simulink model "twoaxis_camera_gantry_start"  (R2021b)
settings: Solver=VariableStepAuto  StartTime=0.0  StopTime=inf  MaxStep=0.01  RelTol=1e-3  AbsTol=0.001  EnableMultiTasking=on
model workspace: external: MATLAB File gantryParams.m (data not in the file)
values from neighbouring files (symbols this model uses):
  endSupport = struct    [gantryParams.m]
  endSupportZ = struct    [gantryParams.m]
  leadScrew = struct    [gantryParams.m]
  leadScrewZ = struct    [gantryParams.m]
  rail = struct    [gantryParams.m]
  railZ = struct    [gantryParams.m]
  runner = struct    [gantryParams.m]
  runnerZ = struct    [gantryParams.m]
undefined symbols (not defined in the file or in its folder): DiscIntNeverNeededParam, X, Y, Z
libraries: sm_lib x81, nesl_utility x30, fl_lib x26, sm_linear_actuator_lib x14, ee_lib x4, slpidlib x2, mspsensorlib x1
(part 1 of 5)
Description:
  | Using the Lead Screw Joint Block - Linear Actuator
  | 
  | This example illustrates the use of the Lead Screw Joint block to model a linear actuator. The Lead
  | Screw Joint block converts rotational motion at the Revolute Joint block to translational motion at
  | the four Cylindrical Joint blocks. The translational motion is specified as a motion input to a
  | cylindrical joint and the necessary actuator torque is automatically computed at the revolute joint.
settings Model: Creator=The MathWorks, Inc.  LastModifiedBy=mligu
settings SolverCC: MaxConsecutiveZCs=100  ZeroCrossAlgorithm=Adaptive  AlgebraicLoopSolver=TrustRegion
settings DataIOCC: SaveFormat=Array  ReturnWorkspaceOutputsName=tp63adcd96_f5aa_4336_8232_618a6ec8fe4f  Refine=20
settings OptimizationCC: LifeSpan=inf
settings DebuggingCC: MaxConsecutiveZCsMsg=none  SolverPrmCheckMsg=warning  AllowSymbolicDim=off  ModelReferenceExtraNoncontSigs=warning  StateNameClashWarn=warning  SFUnexpectedBacktrackingDiag=warning  SFNoUnconditionalDefaultTransitionDiag=warning  SFExecutionAtInitializationDiag=none  SFMachineParentedDataDiag=warning  ArithmeticOperatorsInVariantConditions=warning
settings ModelReferenceCC: PropagateSignalLabelsOutOfModel=off
settings SFSimCC: SimUseLocalCustomCode=off  CustomCodeUndefinedFunction=UseInterfaceOnly
settings RTWCC: RTWUseLocalCustomCode=off
settings CodeAppCC: StateflowObjectComments=on
settings GRTTargetCC: TargetLangStandard=C89/C90 (ANSI)
settings ConfigComp: CovMetricSettings=dw  CovSaveCumulativeToWorkspaceVar=on  CovSaveSingleToWorkspaceVar=on  CovExternalEMLEnable=off  CovSFcnEnable=off
settings SimscapeCC: SimscapeNormalizeSystem=off
settings ConfigurationSet: Description=SimMechanics 2G
settings DiagnosticsConfigSet: SimMechanicsUnconnectedFramePorts=none
settings ExplorerConfigSet: InternalSimMechanicsExplorerSettings="<ExplorerConfiguration><canonicalview>default</canonicalview><AnimationSetting><BasePlaybackSpeed>1.0</BasePlaybackSpeed><PlaybackSpeedFactor>1.0</PlaybackSpeedFactor></AnimationSetting><TilePanel><TileInfo><Tiles Columns=\"1\" Count=\"1\" Rows=\"1\"><Column Weight=\"1\"/><Row Weight=\"1\"/><Tile Height=\"1\" Width=\"1\" X=\"0\" Y=\"0\"/></Tiles></TileInfo><SceneInfo><SceneViewer><BGColor><R>1</R><G>1</G><B>1</B></BGColor><Camera><DoPerspective>off</DoPerspective><Position><X>0.577350260811389404</X><Y>-0.277350261388458308</Y><Z>0.937350262073923357</Z></Position><Center><X>-8.37823641020030152e-09</X><Y>0.300000007801167534</Y><Z>0.35999999288429757</Z></Center><Up><X>-0.408248290463863073</X><Y>0.408248290463863073</Y><Z>0.816496580927726145</Z></Up><ViewLimDist>1</ViewLimDist><YLim>0.483570086956024159</YLim><XLim>0.367001870038164535</XLim></Camera></SceneViewer></SceneInfo></TilePanel><MechEditorPanel><Cameras/><GfxPanelCameraMap/><VideoCreator><PlaybackSpeedRatio>1.0</PlaybackSpeedRatio><FrameRate>30</FrameRate><VideoFormat>Motion JPEG AVI</VideoFormat><FrameSize>auto</FrameSize></VideoCreator></MechEditorPanel></ExplorerConfiguration>"

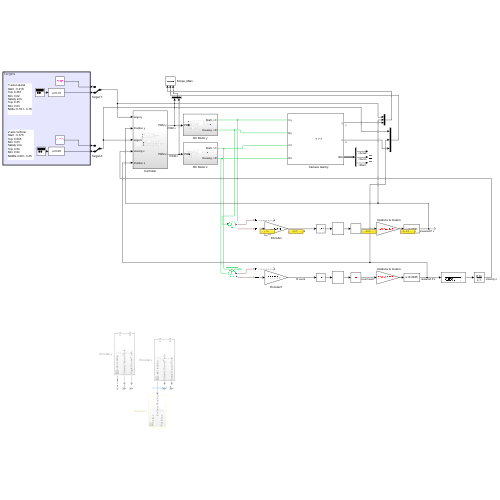
[thumbnail: Simulink's stored preview of the top-level diagram]
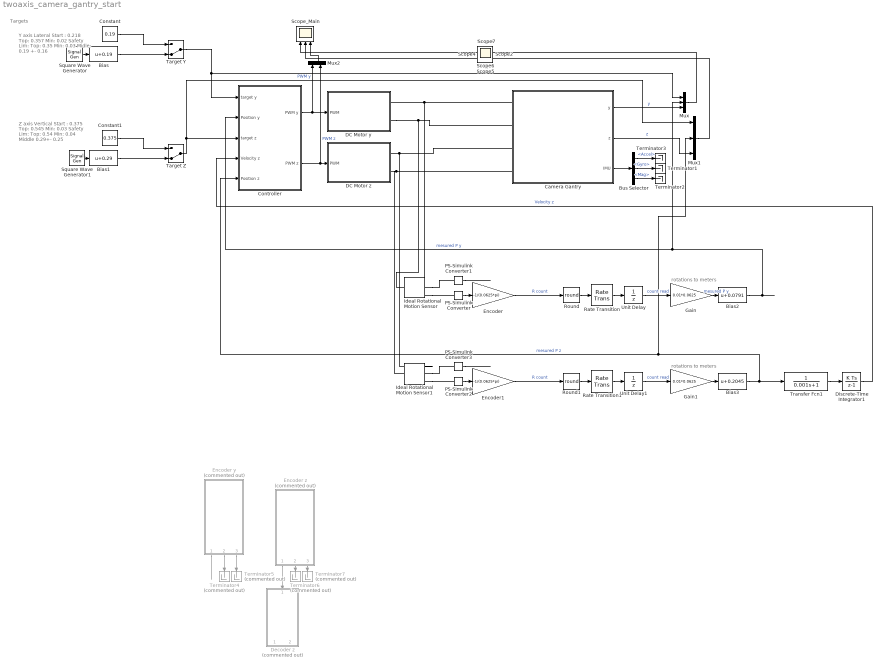
== system twoaxis_camera_gantry_start ==
  note: rotations to meters
  note: Z axis Vertical
      | Start : 0.375
      | Top: 0.545
      | Min: 0.03
      | Safety Lim:
      | Top: 0.54
      | Min: 0.04
      | Middle 0.29+- 0.25
  note: Targets
  note: Y axis Lateral
      | Start : 0.218
      | Top: 0.357
      | Min: 0.02
      | Safety Lim:
      | Top: 0.35
      | Min: 0.03
      | Midle: 0.19 +- 0.16
  note: rotations to meters
  "\tCamera Gantry" : Subsystem
      mask Display: image('C:\Users\cirie\Documents\MCT_labs\coursework_individual\camera_gantry\images\camera_gantry.png'); % Use "Edit Image" on toolstrip to change.
  Bias : Bias  Bias=0.19
  Bias1 : Bias  Bias=0.29
  Bias2 : Bias  Bias=0.0791
  Bias3 : Bias  Bias=0.2045
  Bus Selector : BusSelector  OutputSignals=Accel,Gyro,Mag
  Constant : Constant  Value=0.19
  Constant1 : Constant  Value=0.375
  Controller : Subsystem
  DC Motor y : Subsystem
  DC Motor z : Subsystem
  Decoder z : Subsystem  Commented=on
  Discrete-Time Integrator1 : DiscreteIntegrator  SampleTime=-1  ICPrevOutput=DiscIntNeverNeededParam  ICPrevScaledInput=DiscIntNeverNeededParam
  Encoder : Gain  Gain=-1/(0.0625*pi)
  Encoder y : Subsystem  Commented=on
  Encoder z : Subsystem  Commented=on
  Encoder1 : Gain  Gain=-1/(0.0625*pi)
  Gain : Gain  Gain=0.01*0.0625
  Gain1 : Gain  Gain=0.01*0.0625
  Ideal Rotational Motion Sensor : fl_lib/Mechanical/Mechanical Sensors/Ideal Rotational Motion Sensor  wrap_angle=simscape.enum.onoff.off  offset=0 rad
  Ideal Rotational Motion Sensor1 : fl_lib/Mechanical/Mechanical Sensors/Ideal Rotational Motion Sensor  wrap_angle=simscape.enum.onoff.off  offset=0 rad
  Mux : Mux  Inputs=3
  Mux1 : Mux  Inputs=3
  Mux2 : Mux  Inputs=2
  PS-Simulink Converter{,1..3} (4 alike) : nesl_utility/PS-Simulink Converter  PhysicalDomain=network_engine_domain  SubClassName=ps_output  LeftPortType=input  RightPortType=output  PseudoPeriodic=off  Frequencies=[]  Unit=inherit  AffineConversion=off
      settings: SourceProductBaseCode=PW,SS
  Rate Transition : RateTransition
  Rate Transition1 : RateTransition
  Round : Rounding  Operator=round
  Round1 : Rounding  Operator=round
  Scope_Main : Scope  NumInputPorts=3
  Square Wave Generator : SignalGenerator  Amplitude=0.16  Frequency=0.5  Units=rad/sec
  Square Wave Generator1 : SignalGenerator  Amplitude=0.25  Frequency=0.6  Units=rad/sec
  Target Y : ManualSwitch  CurrentSetting=0
  Target Z : ManualSwitch  CurrentSetting=0
  Terminator1 : Terminator
  Terminator2 : Terminator
  Terminator3 : Terminator
  Terminator{4..7} (4 alike) : Terminator  Commented=on
  Transfer Fcn1 : TransferFcn  Denominator=[0.001 1]
  Unit Delay : UnitDelay  SampleTime=-1  HasFrameUpgradeWarning=on
  Unit Delay1 : UnitDelay  SampleTime=-1  HasFrameUpgradeWarning=on
  Scope{,1..2,4..7} (7 alike) : Scope
  wires:
  "\tCamera Gantry"/3(IMU) -> Bus Selector/1
  Bus Selector/2 -> Terminator1/1  "<Gyro>"
  Bus Selector/3 -> Terminator2/1  "<Mag>"
  "\tCamera Gantry"/2(z) -> Mux1/3  "z"
  Controller/1(PWM y) -> Mux2/1, DC Motor y/1(PWM)  "PWM y"
  Controller/2(PWM z) -> Mux2/2, DC Motor z/1(PWM)  "PWM z"
  Square Wave Generator/1 -> Bias/1
  Square Wave Generator1/1 -> Bias1/1
  Bias/1 -> Target Y/2
  Target Z/1 -> Controller/3(target z), Mux1/1
  Bias1/1 -> Target Z/2
  Constant1/1 -> Target Z/1
  Constant/1 -> Target Y/1
  Target Y/1 -> Controller/1(target y), Mux/1
  Mux/1 -> Scope_Main/1
  Mux1/1 -> Scope_Main/2
  Mux2/1 -> Scope_Main/3
  Bus Selector/1 -> Terminator3/1  "<Accel>"
  Encoder y/1(Encoder reading) -> ?
  Encoder z/1(Encoder reading) -> Decoder z/1(Encoder Reading)
  "\tCamera Gantry"/1(y) -> Mux/3  "y"
  Encoder y/2(Velocity Ground Truth) -> Terminator4/1
  Encoder y/3(Angle Ground Truth) -> Terminator5/1
  Encoder z/2(Velocity Ground Truth) -> Terminator6/1
  Encoder z/3(Angle Ground Truth) -> Terminator7/1
  Bias2/1 -> Controller/2(Position y), Mux/2  "mesured P y"
  Unit Delay/1 -> Gain/1  "count read"
  Encoder/1 -> Round/1  "R count"
  PS-Simulink Converter1/1 -> ?
  Rate Transition/1 -> Unit Delay/1
  Round/1 -> Rate Transition/1
  PS-Simulink Converter/1 -> Encoder/1
  Bias3/1 -> Mux1/2, Controller/5(Position z), Transfer Fcn1/1  "mesured P z"
  Unit Delay1/1 -> Gain1/1  "count read"
  PS-Simulink Converter2/1 -> Encoder1/1
  Encoder1/1 -> Round1/1  "R count"
  Transfer Fcn1/1 -> Discrete-Time Integrator1/1
  PS-Simulink Converter3/1 -> ?
  Round1/1 -> Rate Transition1/1
  Rate Transition1/1 -> Unit Delay1/1
  Discrete-Time Integrator1/1 -> Controller/4(Velocity z)  "Velocity z"
  Gain/1 -> Bias2/1  "mesured P y"
  Gain1/1 -> Bias3/1
  connections:
  "\tCamera Gantry"/LConn3 -- Ideal Rotational Motion Sensor1/RConn1 -- DC Motor z/RConn1
  "\tCamera Gantry"/LConn1 -- Ideal Rotational Motion Sensor/RConn1 -- DC Motor y/RConn1
  DC Motor y/RConn2 -- Ideal Rotational Motion Sensor/LConn1 -- "\tCamera Gantry"/LConn2
  "\tCamera Gantry"/LConn4 -- Ideal Rotational Motion Sensor1/LConn1 -- DC Motor z/RConn2
  Ideal Rotational Motion Sensor/RConn3 -- PS-Simulink Converter/LConn1
  Ideal Rotational Motion Sensor/RConn2 -- PS-Simulink Converter1/LConn1
  Ideal Rotational Motion Sensor1/RConn3 -- PS-Simulink Converter2/LConn1
  Ideal Rotational Motion Sensor1/RConn2 -- PS-Simulink Converter3/LConn1

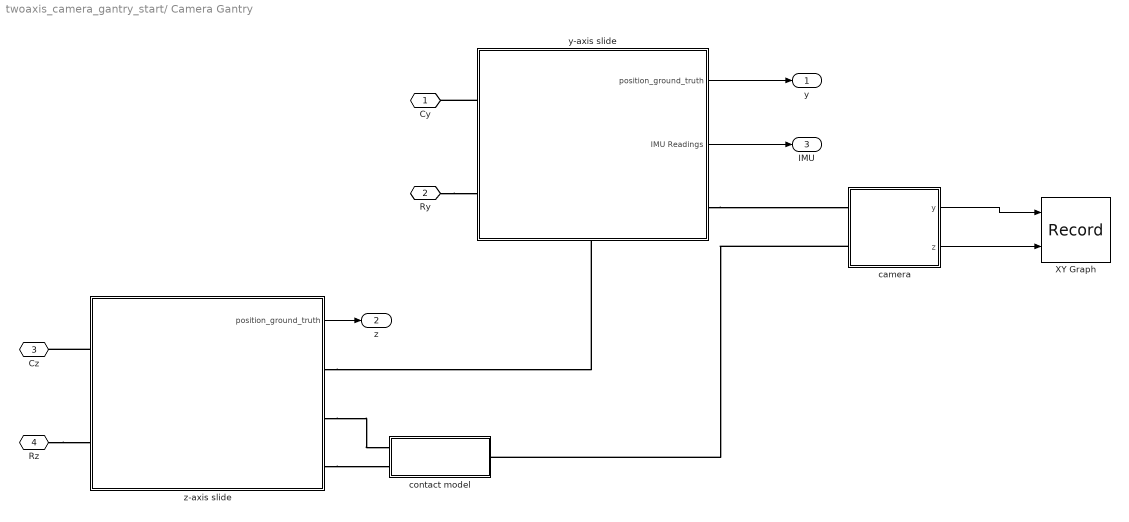
== system twoaxis_camera_gantry_start/	Camera Gantry ==
  XY Graph : Record  FileSettingsInternal="{\"entries\":[{\"content\":{\"excelSettings\":{\"content\":{},\"type\":\"Streamout.ExcelSettings\"}},\"type\":\"Streamout.FileSettingStorage\",\"uuid\":\"845d553e-2d76-460a-b99c-5bdc2b3f34e3\"}],\"packageUris\":[\"http://schema.mathworks.com/mf0/streamout_blocks/R2020a\"],\"version\":\"1.0\"}"  Layout=[1 1]  SignalsInternal="{\"entries\":[{\"content\":{\"signals\":[{\"content\":{\"blockPath\":[\"twoaxis_camera_gantry_start/\\tCamera Gantry/XY Graph\"],\"channel\":[],\"dimensions\":[1],\"domain\":\"twoaxis_camera_gantry_start/\\tCamera Gantry/XY Graph\",\"lineColor\":\"#a2142f\",\"plots\":[1],\"port\":1,\"sid\":[\"\"],\"signalID\":26244,\"signalName\":\"camera:1\"},\"type\":\"RecordBlkView.Signal\",\"uuid\":\"11e20e16-6d29-4cdf-a496-b8ac14960877\"},{\"content\":{\"blockPath\":[\"twoaxis_camera_gantry_start/\\tCamera Gantry/XY Graph\"],\"channel\":[],\"dimensions\":[1],\"domain\":\"twoaxis_camera_gantry_start/\\tCamera Gantry/XY Graph\",\"lineColor\":\"#139fff\",\"plots\":[1],\"port\":2,\"sid\":[\"\"],\"signalID\":26248,\"signalName\":\"camera:2\"},\"type\":\"RecordBlkView.Signal\",\"uuid\":\"c55ae72e-8c87-484c-bada-ad4c492b3dc0\"}]},\"type\":\"RecordBlkView.InputSignals\",\"uuid\":\"5f9b7840-3655-4c14-a584-fe3f6812627c\"}],\"packageUris\":[\"http://schema.mathworks.com/mf0/streamout_blocks/R2020a\"],\"version\":\"1.0\"}"  VisualizationBindings="{\"xyplotplugin\":{\"info\":[{\"series\":[{\"bindingParametersList\":[{\"parameter\":\"X-Axis\",\"signalID\":26244,\"signalName\":\"camera:1\"},{\"parameter\":\"Y-Axis\",\"signalID\":26248,\"signalName\":\"camera:2\"}],\"seriesID\":1443}],\"subplotID\":1}]}}"  CompatibilityTag=XY
  camera : Subsystem
      mask Display: image('$imagefile'); % Use "Edit Image" on toolstrip to change.
  contact model : Subsystem
  y-axis slide : Subsystem
      settings: PortSchema="{\"entries\":[{\"content\":{\"sides\":[{\"content\":{\"connectorIds\":[\"LConn1\",\"LConn2\"]},\"type\":\"ConnectorPlacement.EquallySpacedRectSide\",\"uuid\":\"3f377b63-bc87-4e06-8b63-1d64c166b4f3\"},{\"content\":{\"connectorIds\":[\"Out1\",\"Out2\",\"RConn1\"],\"side\":\"RIGHT\"},\"type\":\"ConnectorPlacement.EquallySpacedRectSide\",\"uuid\":\"3affb14a-8bdc-4f8f-893e-0f417901967e\"},{\"content\":{\"connectorIds\":[],\"side\":\"TOP\"},\"type\":\"ConnectorPlacement.EquallySpacedRectSide\",\"uuid\":\"c82e62d7-ab85-41ce-b1ad-21607245c47e\"},{\"content\":{\"connectorIds\":[\"RConn2\"],\"side\":\"BOTTOM\"},\"type\":\"ConnectorPlacement.EquallySpacedRectSide\",\"uuid\":\"9d54362b-4991-4bea-87e6-d83ba5b68b2b\"}]},\"type\":\"ConnectorPlacement.EquallySpacedConnector\",\"uuid\":\"4017ed31-76af-4f0f-8b41-874461299965\"}],\"packageUris\":[\"http://schema.mathworks.com/mf0/Connector/R2020b\"],\"version\":\"1.0\"}"
      mask Display: image('C:\Users\cirie\Documents\MCT_labs\coursework_individual\camera_gantry\images\slider_rail.png'); % Use "Edit Image" on toolstrip to change.
  z-axis slide : Subsystem
      mask Display: image('C:\Users\cirie\Documents\MCT_labs\coursework_individual\camera_gantry\images\zslider.png'); % Use "Edit Image" on toolstrip to change.
  Cy : PMIOPort  Side=Left
  Ry : PMIOPort  Port=2  Side=Left
  Cz : PMIOPort  Port=3  Side=Left
  Rz : PMIOPort  Port=4  Side=Left
  y : Outport
  z : Outport  Port=2
  IMU : Outport  Port=3
  wires:
  camera/1(y) -> XY Graph/1
  y-axis slide/1(position_ground_truth) -> y/1
  y-axis slide/2(IMU Readings) -> IMU/1
  z-axis slide/1(position_ground_truth) -> z/1
  camera/2(z) -> XY Graph/2
  connections:
  y-axis slide/LConn1 -- Cy/RConn1
  Ry/RConn1 -- y-axis slide/LConn2
  y-axis slide/RConn1 -- camera/LConn1
  z-axis slide/LConn1 -- Cz/RConn1
  Rz/RConn1 -- z-axis slide/LConn2
  z-axis slide/RConn1 -- y-axis slide/RConn2
  z-axis slide/RConn2 -- contact model/LConn1
  z-axis slide/RConn3 -- contact model/LConn2
  camera/LConn2 -- contact model/RConn1

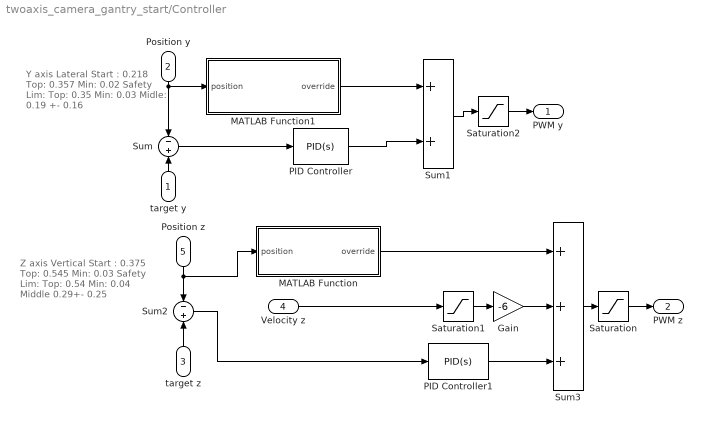
== system twoaxis_camera_gantry_start/Controller ==
  note: Y axis Lateral
      | Start : 0.218
      | Top: 0.357
      | Min: 0.02
      | Safety Lim:
      | Top: 0.35
      | Min: 0.03
      | Midle: 0.19 +- 0.16
  note: Z axis Vertical
      | Start : 0.375
      | Top: 0.545
      | Min: 0.03
      | Safety Lim:
      | Top: 0.54
      | Min: 0.04
      | Middle 0.29+- 0.25
  target y : Inport
  Position y : Inport  Port=2
  target z : Inport  Port=3
  Velocity z : Inport  Port=4
  Position z : Inport  Port=5
  Gain : Gain  Gain=-6
  MATLAB Function : MATLAB Function  TreatAsAtomicUnit=on
  MATLAB Function1 : MATLAB Function  TreatAsAtomicUnit=on
  PID Controller : slpidlib/PID Controller  Controller=PID  Form=Parallel  TimeDomain=Continuous-time  UseExternalTs=off  SampleTime=-1  IntegratorMethod=Forward Euler  FilterMethod=Forward Euler  ControllerParametersSource=internal  P=300  I=1  D=10  UseFilter=on  N=100  TunerSelectOption=Transfer Function Based (PID Tuner App)  InitialConditionSource=internal  InitialConditionForIntegrator=0  InitialConditionForFilter=0  DifferentiatorICPrevScaledInput=0  ExternalReset=none  TrackingMode=off  Kt=1  LimitOutput=on  SatLimitsSource=internal  UpperSaturationLimit=1  LowerSaturationLimit=-1  LinearizeAsGain=on  AntiWindupMode=none  Kb=1  POutMin=[]  POutMax=[]  IOutMin=[]  IOutMax=[]  DOutMin=[]  DOutMax=[]  NOutMin=[]  NOutMax=[]  SumOutMin=[]  SumOutMax=[]  SaturationOutMin=[]  SaturationOutMax=[]  PParamMin=[]  PParamMax=[]  IParamMin=[]  IParamMax=[]  DParamMin=[]  DParamMax=[]  NParamMin=[]  NParamMax=[]  KbParamMin=[]  KbParamMax=[]  KtParamMin=[]  KtParamMax=[]  KbOutMin=[]  KbOutMax=[]  KtOutMin=[]  KtOutMax=[]  IntegratorOutMin=[]  IntegratorOutMax=[]  FilterOutMin=[]  FilterOutMax=[]  SumI1OutMin=[]  SumI1OutMax=[]  SumI2OutMin=[]  SumI2OutMax=[]  SumI3OutMin=[]  SumI3OutMax=[]  SumI4OutMin=[]  SumI4OutMax=[]  SumDOutMin=[]  SumDOutMax=[]  DifferentiatorOutMin=[]  DifferentiatorOutMax=[]  FilterDiffOutCoefMin=[]  FilterDiffOutCoefMax=[]  ReciprocalOutMin=[]  ReciprocalOutMax=[]  SumDenOutMin=[]  SumDenOutMax=[]  SumNumOutMin=[]  SumNumOutMax=[]  DivideOutMin=[]  DivideOutMax=[]  UdiffTsProdOutMin=[]  UdiffTsProdOutMax=[]  NTsProdOutMin=[]  NTsProdOutMax=[]  UintegralTsProdOutMin=[]  UintegralTsProdOutMax=[]  UngainTsProdOutMin=[]  UngainTsProdOutMax=[]  IntegratorContinuousStateAttributes=''  IntegratorStateMustResolveToSignalObject=off  IntegratorRTWStateStorageClass=Auto  FilterContinuousStateAttributes=''  FilterStateMustResolveToSignalObject=off  FilterRTWStateStorageClass=Auto  ParallelPVariant=InternalParameters  IdealPVariant=Disabled  IVariant=InternalParameters  DVariant=InternalParameters  IntegratorVariant=Continuous  SatVariant=Enabled  AWVariant=Passthrough  PCopyVariant=Disabled  TRVariant=Disabled  FdbkBlocksVariant=Forward  IdealPFdbkVariant=Disabled  SatFdbkVariant=Disabled  DerivativeFilterVariant=ContFilter  NVariant=InternalParameters  NCopyVariant=Disabled  FilterICVariant=InternalICsFilter  IntegratorICVariant=InternalICs  ExternalResetVariant=Disabled  TRSumVariant=Passthrough  SumFdbkVariant=Disabled  SumVariant=Sum_PID  TsampFilterVariant=InternalTs  TsampNgainVariant=Passthrough  TsampIntegralVariant=Passthrough  ExternalSaturationOutDataTypeStr=Inherit: Same as second input
  PID Controller1 : slpidlib/PID Controller  Controller=PID  Form=Parallel  TimeDomain=Continuous-time  UseExternalTs=off  SampleTime=-1  IntegratorMethod=Forward Euler  FilterMethod=Forward Euler  ControllerParametersSource=internal  P=300  I=0  D=10  UseFilter=on  N=100  TunerSelectOption=Transfer Function Based (PID Tuner App)  InitialConditionSource=internal  InitialConditionForIntegrator=0  InitialConditionForFilter=0  DifferentiatorICPrevScaledInput=0  ExternalReset=none  TrackingMode=off  Kt=1  LimitOutput=on  SatLimitsSource=internal  UpperSaturationLimit=1  LowerSaturationLimit=-1  LinearizeAsGain=on  AntiWindupMode=none  Kb=1  POutMin=[]  POutMax=[]  IOutMin=[]  IOutMax=[]  DOutMin=[]  DOutMax=[]  NOutMin=[]  NOutMax=[]  SumOutMin=[]  SumOutMax=[]  SaturationOutMin=[]  SaturationOutMax=[]  PParamMin=[]  PParamMax=[]  IParamMin=[]  IParamMax=[]  DParamMin=[]  DParamMax=[]  NParamMin=[]  NParamMax=[]  KbParamMin=[]  KbParamMax=[]  KtParamMin=[]  KtParamMax=[]  KbOutMin=[]  KbOutMax=[]  KtOutMin=[]  KtOutMax=[]  IntegratorOutMin=[]  IntegratorOutMax=[]  FilterOutMin=[]  FilterOutMax=[]  SumI1OutMin=[]  SumI1OutMax=[]  SumI2OutMin=[]  SumI2OutMax=[]  SumI3OutMin=[]  SumI3OutMax=[]  SumI4OutMin=[]  SumI4OutMax=[]  SumDOutMin=[]  SumDOutMax=[]  DifferentiatorOutMin=[]  DifferentiatorOutMax=[]  FilterDiffOutCoefMin=[]  FilterDiffOutCoefMax=[]  ReciprocalOutMin=[]  ReciprocalOutMax=[]  SumDenOutMin=[]  SumDenOutMax=[]  SumNumOutMin=[]  SumNumOutMax=[]  DivideOutMin=[]  DivideOutMax=[]  UdiffTsProdOutMin=[]  UdiffTsProdOutMax=[]  NTsProdOutMin=[]  NTsProdOutMax=[]  UintegralTsProdOutMin=[]  UintegralTsProdOutMax=[]  UngainTsProdOutMin=[]  UngainTsProdOutMax=[]  IntegratorContinuousStateAttributes=''  IntegratorStateMustResolveToSignalObject=off  IntegratorRTWStateStorageClass=Auto  FilterContinuousStateAttributes=''  FilterStateMustResolveToSignalObject=off  FilterRTWStateStorageClass=Auto  ParallelPVariant=InternalParameters  IdealPVariant=Disabled  IVariant=InternalParameters  DVariant=InternalParameters  IntegratorVariant=Continuous  SatVariant=Enabled  AWVariant=Passthrough  PCopyVariant=Disabled  TRVariant=Disabled  FdbkBlocksVariant=Forward  IdealPFdbkVariant=Disabled  SatFdbkVariant=Disabled  DerivativeFilterVariant=ContFilter  NVariant=InternalParameters  NCopyVariant=Disabled  FilterICVariant=InternalICsFilter  IntegratorICVariant=InternalICs  ExternalResetVariant=Disabled  TRSumVariant=Passthrough  SumFdbkVariant=Disabled  SumVariant=Sum_PID  TsampFilterVariant=InternalTs  TsampNgainVariant=Passthrough  TsampIntegralVariant=Passthrough  ExternalSaturationOutDataTypeStr=Inherit: Same as second input
  Saturation : Saturate  UpperLimit=1  LowerLimit=-1
  Saturation1 : Saturate  UpperLimit=0  LowerLimit=-10
  Saturation2 : Saturate  UpperLimit=1  LowerLimit=-1
  Sum : Sum  Inputs=-|+
  Sum1 : Sum
  Sum2 : Sum  Inputs=-|+
  Sum3 : Sum  Inputs=+++
  PWM y : Outport
  PWM z : Outport  Port=2
  wires:
  Sum/1 -> PID Controller/1
  target y/1 -> Sum/2
  Sum2/1 -> PID Controller1/1
  target z/1 -> Sum2/2
  PID Controller/1 -> Sum1/2
  Sum3/1 -> Saturation/1
  Saturation1/1 -> Gain/1
  Saturation/1 -> PWM z/1
  Gain/1 -> Sum3/2
  Sum1/1 -> Saturation2/1
  Saturation2/1 -> PWM y/1
  Position y/1 -> Sum/1, MATLAB Function1/1(position)
  MATLAB Function1/1(override) -> Sum1/1
  PID Controller1/1 -> Sum3/3
  MATLAB Function/1(override) -> Sum3/1
  Position z/1 -> Sum2/1, MATLAB Function/1(position)
  Velocity z/1 -> Saturation1/1

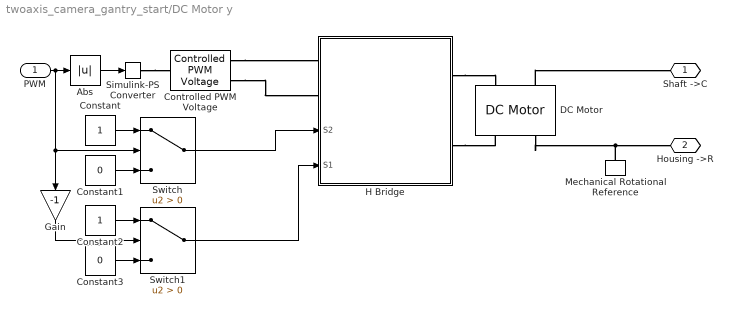
== system twoaxis_camera_gantry_start/DC Motor y ==
  PWM : Inport
  Abs : Abs
  Constant : Constant
  Constant1 : Constant  Value=0
  Constant2 : Constant
  Constant3 : Constant  Value=0
  Controlled PWM Voltage : ee_lib/Integrated Circuits/Controlled PWM Voltage  F=5000 Hz  TD=0 s  pulse_width_offset=0 s  pulse_min=0 s  pwm_or_av=2  event_type=1  sample_time=1e-6 s  Vmin=0 V  Vmax=5 V  Vm=12 V  u_min=0  u_max=1
      settings: InternalSimscapePortConfiguration="{\"Bottom\":[],\"Left\":[{\"id\":\"u\",\"label\":\"u\",\"type\":\"input\"}],\"Right\":[{\"id\":\"p2\",\"label\":\"PWM\",\"type\":\"foundation.electrical.electrical\"},{\"id\":\"n2\",\"label\":\"REF\",\"type\":\"foundation.electrical.electrical\"}],\"Top\":[]}"
  DC Motor : ee_lib/Electromechanical/Brushed Motors/DC Motor  field_option=ee.enum.field_option.pm  Rf=100 Ohm  Lf=1 H  Laf=0.15 H  If0=0 A  parameterization=ee.enum.dcparam_option.load_speed  Ra=3.9 Ohm  La=12e-6 H  emf_or_torque=ee.enum.emf_or_torque.kv  Kv=0.072e-3 V/rpm  Ki=6.876e-4 N*m/A  T_stall="0.04903325  N*m"  w_max=19100 rpm  w_rated=15000 rpm  P_rated=100 W  V_rated=12 V  lam_param=ee.enum.lam_param.damping  i_noload=0 A  V_i_noload=1.5 V  J=0.01 g*cm^2  lam=0 N*m/(rad/s)  speed0=0 rpm  enable_fault_armature=simscape.enum.onoff.off  rev_faulted=1 / 3  G_faulted_armature=1e-5 S  fault_trigger_armature=ee.enum.faults.faultTrigger.temporal  t_fault_armature=1 s  max_permissible_current_armature=inf A  t_fail_on_current_armature=1 s  enable_fault_field=simscape.enum.onoff.off  G_faulted_field=1e-5 S  fault_trigger_field=ee.enum.faults.faultTrigger.temporal  t_fault_field=1 s  max_permissible_current_field=inf A  t_fail_on_current_field=1 s  fault_action=simscape.enum.assert.action.none  alpha=3.93e-3 1/K  Tmeas=25 degC  thermal_mass=100 J/K  initial_temperature=25 degC
  Gain : Gain  Gain=-1
  H Bridge : Subsystem
      settings: PortSchema="{\"entries\":[{\"content\":{\"sides\":[{\"content\":{\"connectorIds\":[\"LConn1\",\"LConn2\",\"In1\",\"In2\"]},\"type\":\"ConnectorPlacement.EquallySpacedRectSide\",\"uuid\":\"c8ec8bc9-4623-4c55-ab9b-87835642b339\"},{\"content\":{\"connectorIds\":[\"RConn1\",\"RConn2\"],\"side\":\"RIGHT\"},\"type\":\"ConnectorPlacement.EquallySpacedRectSide\",\"uuid\":\"7c39eb40-a15c-4472-a1f8-12def0cf9357\"},{\"content\":{\"connectorIds\":[],\"side\":\"TOP\"},\"type\":\"ConnectorPlacement.EquallySpacedRectSide\",\"uuid\":\"b7d11f50-d295-4c56-a5c2-c3a41b45caf9\"},{\"content\":{\"connectorIds\":[],\"side\":\"BOTTOM\"},\"type\":\"ConnectorPlacement.EquallySpacedRectSide\",\"uuid\":\"50bd01d5-9f64-4ab9-b8fc-fcc3feacf34c\"}]},\"type\":\"ConnectorPlacement.EquallySpacedConnector\",\"uuid\":\"92be81d0-1e08-4b05-b26c-58c06fe84849\"}],\"packageUris\":[\"http://schema.mathworks.com/mf0/Connector/R2020b\"],\"version\":\"1.0\"}"
      mask Display: image(imread('SN_H_Bridge.jpg'));
  Mechanical Rotational Reference : fl_lib/Mechanical/Rotational Elements/Mechanical Rotational Reference
  Simulink-PS Converter : nesl_utility/Simulink-PS Converter  PhysicalDomain=network_engine_domain  SubClassName=ps_input  LeftPortType=input  RightPortType=output  PseudoPeriodic=off  Frequencies=[]  NoiseDistribution=none  NoiseParameters=[]  Unit=1  AffineConversion=off  FilteringAndDerivatives=provide  SimscapeFilterOrder=1  InputFilterTimeConstant=0.001  UdotUserProvided=0
      settings: SourceProductBaseCode=PW,SS
  Switch : Switch  Criteria=u2 > Threshold
  Switch1 : Switch  Criteria=u2 > Threshold
  Shaft ->C : PMIOPort  Side=Right
  Housing ->R : PMIOPort  Port=2  Side=Right
  wires:
  Switch/1 -> H Bridge/1(S2)
  Switch1/1 -> H Bridge/2(S1)
  Abs/1 -> Simulink-PS Converter/1
  Constant1/1 -> Switch/3
  Gain/1 -> Switch1/2
  Constant/1 -> Switch/1
  Constant3/1 -> Switch1/3
  Constant2/1 -> Switch1/1
  PWM/1 -> Gain/1, Switch/2, Abs/1
  connections:
  Mechanical Rotational Reference/LConn1 -- DC Motor/RConn2 -- Housing ->R/RConn1
  DC Motor/LConn2 -- Shaft ->C/RConn1
  Simulink-PS Converter/RConn1 -- Controlled PWM Voltage/LConn1
  H Bridge/RConn1 -- DC Motor/LConn1
  H Bridge/RConn2 -- DC Motor/RConn1
  Controlled PWM Voltage/RConn1 -- H Bridge/LConn1
  Controlled PWM Voltage/RConn2 -- H Bridge/LConn2

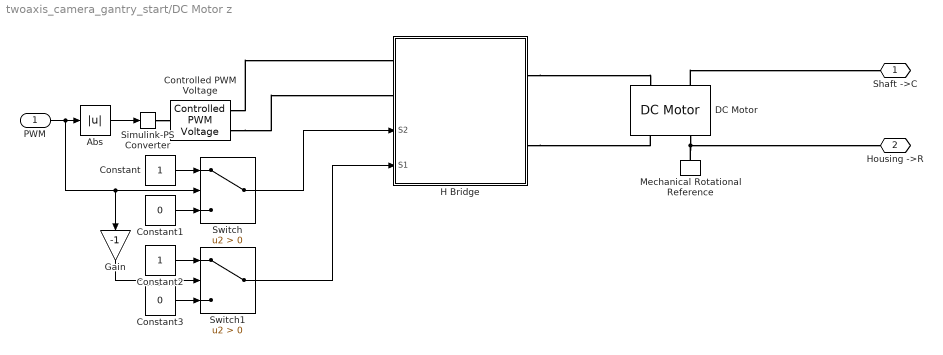
== system twoaxis_camera_gantry_start/DC Motor z ==
  PWM : Inport
  Abs : Abs
  Constant : Constant
  Constant1 : Constant  Value=0
  Constant2 : Constant
  Constant3 : Constant  Value=0
  Controlled PWM Voltage : ee_lib/Integrated Circuits/Controlled PWM Voltage  F=5000 Hz  TD=0 s  pulse_width_offset=0 s  pulse_min=0 s  pwm_or_av=2  event_type=1  sample_time=1e-6 s  Vmin=0 V  Vmax=5 V  Vm=12 V  u_min=0  u_max=1
      settings: InternalSimscapePortConfiguration="{\"Bottom\":[],\"Left\":[{\"id\":\"u\",\"label\":\"u\",\"type\":\"input\"}],\"Right\":[{\"id\":\"p2\",\"label\":\"PWM\",\"type\":\"foundation.electrical.electrical\"},{\"id\":\"n2\",\"label\":\"REF\",\"type\":\"foundation.electrical.electrical\"}],\"Top\":[]}"
  DC Motor : ee_lib/Electromechanical/Brushed Motors/DC Motor  field_option=ee.enum.field_option.pm  Rf=100 Ohm  Lf=1 H  Laf=0.15 H  If0=0 A  parameterization=ee.enum.dcparam_option.load_speed  Ra=3.9 Ohm  La=12e-6 H  emf_or_torque=ee.enum.emf_or_torque.kv  Kv=0.072e-3 V/rpm  Ki=6.876e-4 N*m/A  T_stall="0.04903325  N*m"  w_max=19100 rpm  w_rated=15000 rpm  P_rated=100 W  V_rated=12 V  lam_param=ee.enum.lam_param.damping  i_noload=0 A  V_i_noload=1.5 V  J=0.01 g*cm^2  lam=0 N*m/(rad/s)  speed0=0 rpm  enable_fault_armature=simscape.enum.onoff.off  rev_faulted=1 / 3  G_faulted_armature=1e-5 S  fault_trigger_armature=ee.enum.faults.faultTrigger.temporal  t_fault_armature=1 s  max_permissible_current_armature=inf A  t_fail_on_current_armature=1 s  enable_fault_field=simscape.enum.onoff.off  G_faulted_field=1e-5 S  fault_trigger_field=ee.enum.faults.faultTrigger.temporal  t_fault_field=1 s  max_permissible_current_field=inf A  t_fail_on_current_field=1 s  fault_action=simscape.enum.assert.action.none  alpha=3.93e-3 1/K  Tmeas=25 degC  thermal_mass=100 J/K  initial_temperature=25 degC
  Gain : Gain  Gain=-1
  H Bridge : Subsystem
      settings: PortSchema="{\"entries\":[{\"content\":{\"sides\":[{\"content\":{\"connectorIds\":[\"LConn1\",\"LConn2\",\"In1\",\"In2\"]},\"type\":\"ConnectorPlacement.EquallySpacedRectSide\",\"uuid\":\"c8ec8bc9-4623-4c55-ab9b-87835642b339\"},{\"content\":{\"connectorIds\":[\"RConn1\",\"RConn2\"],\"side\":\"RIGHT\"},\"type\":\"ConnectorPlacement.EquallySpacedRectSide\",\"uuid\":\"7c39eb40-a15c-4472-a1f8-12def0cf9357\"},{\"content\":{\"connectorIds\":[],\"side\":\"TOP\"},\"type\":\"ConnectorPlacement.EquallySpacedRectSide\",\"uuid\":\"b7d11f50-d295-4c56-a5c2-c3a41b45caf9\"},{\"content\":{\"connectorIds\":[],\"side\":\"BOTTOM\"},\"type\":\"ConnectorPlacement.EquallySpacedRectSide\",\"uuid\":\"50bd01d5-9f64-4ab9-b8fc-fcc3feacf34c\"}]},\"type\":\"ConnectorPlacement.EquallySpacedConnector\",\"uuid\":\"92be81d0-1e08-4b05-b26c-58c06fe84849\"}],\"packageUris\":[\"http://schema.mathworks.com/mf0/Connector/R2020b\"],\"version\":\"1.0\"}"
      mask Display: image(imread('SN_H_Bridge.jpg'));
  Mechanical Rotational Reference : fl_lib/Mechanical/Rotational Elements/Mechanical Rotational Reference
  Simulink-PS Converter : nesl_utility/Simulink-PS Converter  PhysicalDomain=network_engine_domain  SubClassName=ps_input  LeftPortType=input  RightPortType=output  PseudoPeriodic=off  Frequencies=[]  NoiseDistribution=none  NoiseParameters=[]  Unit=1  AffineConversion=off  FilteringAndDerivatives=provide  SimscapeFilterOrder=1  InputFilterTimeConstant=0.001  UdotUserProvided=0
      settings: SourceProductBaseCode=PW,SS
  Switch : Switch  Criteria=u2 > Threshold
  Switch1 : Switch  Criteria=u2 > Threshold
  Shaft ->C : PMIOPort  Side=Right
  Housing ->R : PMIOPort  Port=2  Side=Right
  wires:
  Switch/1 -> H Bridge/1(S2)
  Switch1/1 -> H Bridge/2(S1)
  Abs/1 -> Simulink-PS Converter/1
  Constant1/1 -> Switch/3
  Gain/1 -> Switch1/2
  Constant/1 -> Switch/1
  Constant3/1 -> Switch1/3
  Constant2/1 -> Switch1/1
  PWM/1 -> Gain/1, Switch/2, Abs/1
  connections:
  Mechanical Rotational Reference/LConn1 -- DC Motor/RConn2 -- Housing ->R/RConn1
  DC Motor/LConn2 -- Shaft ->C/RConn1
  Simulink-PS Converter/RConn1 -- Controlled PWM Voltage/LConn1
  H Bridge/RConn1 -- DC Motor/LConn1
  H Bridge/RConn2 -- DC Motor/RConn1
  Controlled PWM Voltage/RConn1 -- H Bridge/LConn1
  Controlled PWM Voltage/RConn2 -- H Bridge/LConn2

== system twoaxis_camera_gantry_start/Decoder z ==
  Encoder Reading : Inport
  Discrete-Time Integrator : DiscreteIntegrator  SampleTime=-1  ICPrevOutput=DiscIntNeverNeededParam  ICPrevScaledInput=DiscIntNeverNeededParam
  Gain : Gain  Gain=2*pi/(2^5)
  Transfer Fcn : TransferFcn  Denominator=[0.001 1]
  Velocity z : Outport
  Position z : Outport  Port=2
  wires:
  Gain/1 -> Position z/1, Transfer Fcn/1
  Encoder Reading/1 -> Gain/1
  Transfer Fcn/1 -> Discrete-Time Integrator/1
  Discrete-Time Integrator/1 -> Velocity z/1

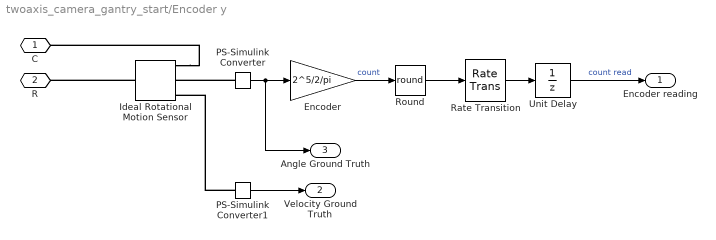
== system twoaxis_camera_gantry_start/Encoder y ==
  Encoder : Gain  Gain=2^5/2/pi
  Ideal Rotational Motion Sensor : fl_lib/Mechanical/Mechanical Sensors/Ideal Rotational Motion Sensor  wrap_angle=simscape.enum.onoff.off  offset=0 rad
  PS-Simulink Converter : nesl_utility/PS-Simulink Converter  PhysicalDomain=network_engine_domain  SubClassName=ps_output  LeftPortType=input  RightPortType=output  PseudoPeriodic=off  Frequencies=[]  Unit=inherit  AffineConversion=off
      settings: SourceProductBaseCode=PW,SS
  PS-Simulink Converter1 : nesl_utility/PS-Simulink Converter  PhysicalDomain=network_engine_domain  SubClassName=ps_output  LeftPortType=input  RightPortType=output  PseudoPeriodic=off  Frequencies=[]  Unit=inherit  AffineConversion=off
      settings: SourceProductBaseCode=PW,SS
  Rate Transition : RateTransition
  Round : Rounding  Operator=round
  Unit Delay : UnitDelay  SampleTime=-1  HasFrameUpgradeWarning=on
  C : PMIOPort  Side=Left
  R : PMIOPort  Port=2  Side=Left
  Encoder reading : Outport
  Velocity Ground Truth : Outport  Port=2
  Angle Ground Truth : Outport  Port=3
  wires:
  Round/1 -> Rate Transition/1
  Rate Transition/1 -> Unit Delay/1
  PS-Simulink Converter1/1 -> Velocity Ground Truth/1
  Encoder/1 -> Round/1  "count"
  PS-Simulink Converter/1 -> Angle Ground Truth/1, Encoder/1
  Unit Delay/1 -> Encoder reading/1  "count read"
  connections:
  PS-Simulink Converter/LConn1 -- Ideal Rotational Motion Sensor/RConn2
  Ideal Rotational Motion Sensor/LConn1 -- R/RConn1
  PS-Simulink Converter1/LConn1 -- Ideal Rotational Motion Sensor/RConn3
  Ideal Rotational Motion Sensor/RConn1 -- C/RConn1

== system twoaxis_camera_gantry_start/Encoder z ==
  Encoder : Gain  Gain=2^5/2/pi
  Ideal Rotational Motion Sensor : fl_lib/Mechanical/Mechanical Sensors/Ideal Rotational Motion Sensor  wrap_angle=simscape.enum.onoff.off  offset=0 rad
  PS-Simulink Converter : nesl_utility/PS-Simulink Converter  PhysicalDomain=network_engine_domain  SubClassName=ps_output  LeftPortType=input  RightPortType=output  PseudoPeriodic=off  Frequencies=[]  Unit=inherit  AffineConversion=off
      settings: SourceProductBaseCode=PW,SS
  PS-Simulink Converter1 : nesl_utility/PS-Simulink Converter  PhysicalDomain=network_engine_domain  SubClassName=ps_output  LeftPortType=input  RightPortType=output  PseudoPeriodic=off  Frequencies=[]  Unit=inherit  AffineConversion=off
      settings: SourceProductBaseCode=PW,SS
  Rate Transition : RateTransition
  Round : Rounding  Operator=round
  Unit Delay : UnitDelay  SampleTime=-1  HasFrameUpgradeWarning=on
  C : PMIOPort  Side=Left
  R : PMIOPort  Port=2  Side=Left
  Encoder reading : Outport
  Velocity Ground Truth : Outport  Port=2
  Angle Ground Truth : Outport  Port=3
  wires:
  Round/1 -> Rate Transition/1
  Rate Transition/1 -> Unit Delay/1
  PS-Simulink Converter1/1 -> Velocity Ground Truth/1
  Encoder/1 -> Round/1  "count"
  PS-Simulink Converter/1 -> Angle Ground Truth/1, Encoder/1
  Unit Delay/1 -> Encoder reading/1  "count read"
  connections:
  PS-Simulink Converter/LConn1 -- Ideal Rotational Motion Sensor/RConn2
  Ideal Rotational Motion Sensor/LConn1 -- R/RConn1
  PS-Simulink Converter1/LConn1 -- Ideal Rotational Motion Sensor/RConn3
  Ideal Rotational Motion Sensor/RConn1 -- C/RConn1

== system twoaxis_camera_gantry_start/	Camera Gantry/camera ==
  File Solid : sm_lib/Body Elements/File Solid  ExtGeomFileName=canon.stl  UnitType=Custom  ExtGeomFileUnits=mm  StepReaderType=HEX  ExportConvexHullGeometry=on  InertiaType=CalculateFromGeometry  Mass=1  MassUnits=kg  CenterOfMass=[0 0 0]  CenterOfMassUnits=m  MomentsOfInertia=[1 1 1]  MomentsOfInertiaUnits=kg*m^2  ProductsOfInertia=[0 0 0]  ProductsOfInertiaUnits=kg*m^2  BasedOnType=Density  Density=0.72  DensityUnits=g/cm^3  DoExposeReferenceFrame=off  SerializedFrames=<Frames><Frame><Id>Frame1</Id><Value><Name>F1</Name><Origin><Source>CenterOfMassFrame</Source><FeatureName></FeatureName></Origin><PrimaryAxis><DefinedDirection>+Z</DefinedDirection><Source>ReferenceFrame</Source><SourceDirection>+Z</SourceDirection><FeatureName></FeatureName></PrimaryAxis><SecondaryAxis><DefinedDirection>+X</DefinedDirection><Source>ReferenceFrame</Source><SourceDirection>+X</SourceDirection><FeatureName></FeatureName></SecondaryAxis></Value></Frame></Frames>  GraphicType=FromGeometry  MarkerShape=Sphere  MarkerSize=10  GraphicVisPropType=SimpleVisualProperties  GraphicDiffuseColor=[0.5 0.5 0.5]  GraphicSpecularColor=[0.5 0.5 0.5 1.0]  GraphicAmbientColor=[0.15 0.15 0.15 1.0]  GraphicEmissiveColor=[0.0 0.0 0.0 1.0]  GraphicShininess=75  GraphicOpacity=1.0
  PS-Simulink Converter : nesl_utility/PS-Simulink Converter  PhysicalDomain=network_engine_domain  SubClassName=ps_output  LeftPortType=input  RightPortType=output  PseudoPeriodic=off  Frequencies=[]  Unit=inherit  AffineConversion=off
      settings: SourceProductBaseCode=PW,SS
  PS-Simulink Converter1 : nesl_utility/PS-Simulink Converter  PhysicalDomain=network_engine_domain  SubClassName=ps_output  LeftPortType=input  RightPortType=output  PseudoPeriodic=off  Frequencies=[]  Unit=inherit  AffineConversion=off
      settings: SourceProductBaseCode=PW,SS
  Rigid Transform : sm_lib/Frames and Transforms/Rigid Transform  TranslationMethod=None  TranslationStandardOffset=0  TranslationLengthUnit=m  TranslationStandardAxis=+Z  TranslationCartesianOffset=[0 0 0]  TranslationROffset=0  TranslationROffsetUnits=m  TranslationZOffset=0  TranslationZOffsetUnits=m  TranslationThetaOffset=0  TranslationThetaOffsetUnits=deg  RotationMethod=StandardAxis  RotationAngleUnits=deg  RotationStandardAxis=-X  RotationAngle=90  RotationArbitraryAxis=[0 0 1]  FollAlignAxisA=+X  BaseAlignAxisA=+Y  FollAlignAxisB=+Y  BaseAlignAxisB=+Z  RotationSequenceAxes=FollowerAxes  RotationSequence=XYX  RotationSequenceAngles=[0 0 0]  RotationSequenceAnglesUnits=deg  RotationMatrix=[1 0 0; 0 1 0; 0 0 1]
  Rigid Transform1 : sm_lib/Frames and Transforms/Rigid Transform  TranslationMethod=None  TranslationStandardOffset=0  TranslationLengthUnit=m  TranslationStandardAxis=+Z  TranslationCartesianOffset=[0 0 0]  TranslationROffset=0  TranslationROffsetUnits=m  TranslationZOffset=0  TranslationZOffsetUnits=m  TranslationThetaOffset=0  TranslationThetaOffsetUnits=deg  RotationMethod=StandardAxis  RotationAngleUnits=deg  RotationStandardAxis=+Z  RotationAngle=90  RotationArbitraryAxis=[0 0 1]  FollAlignAxisA=+X  BaseAlignAxisA=+Y  FollAlignAxisB=+Y  BaseAlignAxisB=+Z  RotationSequenceAxes=FollowerAxes  RotationSequence=XYX  RotationSequenceAngles=[0 0 0]  RotationSequenceAnglesUnits=deg  RotationMatrix=[1 0 0; 0 1 0; 0 0 1]
  Rigid Transform2 : sm_lib/Frames and Transforms/Rigid Transform  TranslationMethod=Cartesian  TranslationStandardOffset=47  TranslationLengthUnit=mm  TranslationStandardAxis=+Z  TranslationCartesianOffset=[0 -30 47]  TranslationROffset=0  TranslationROffsetUnits=m  TranslationZOffset=0  TranslationZOffsetUnits=m  TranslationThetaOffset=0  TranslationThetaOffsetUnits=deg  RotationMethod=None  RotationAngleUnits=deg  RotationStandardAxis=+Z  RotationAngle=90  RotationArbitraryAxis=[0 0 1]  FollAlignAxisA=+X  BaseAlignAxisA=+Y  FollAlignAxisB=+Y  BaseAlignAxisB=+Z  RotationSequenceAxes=FollowerAxes  RotationSequence=XYX  RotationSequenceAngles=[0 0 0]  RotationSequenceAnglesUnits=deg  RotationMatrix=[1 0 0; 0 1 0; 0 0 1]
  Transform Sensor : sm_lib/Frames and Transforms/Transform Sensor  MeasurementFrame=World  SenseAngle=off  SenseAxis=off  SenseAngle1=off  SenseAngle2=off  SenseAngle3=off  SenseQ=off  SenseR=off  SenseOmegaX=off  SenseOmegaY=off  SenseOmegaZ=off  SenseOmega1=off  SenseOmega2=off  SenseOmega3=off  SenseQDot=off  SenseRDot=off  SenseAlphaX=off  SenseAlphaY=off  SenseAlphaZ=off  SenseAlpha1=off  SenseAlpha2=off  SenseAlpha3=off  SenseQDDot=off  SenseRDDot=off  SenseX=off  SenseY=on  SenseZ=on  SenseRad=off  SenseAzim=off  SenseDist=off  SenseInc=off  SenseXDot=off  SenseYDot=off  SenseZDot=off  SenseRadDot=off  SenseAzimDot=off  SenseDistDot=off  SenseIncDot=off  SenseXDDot=off  SenseYDDot=off  SenseZDDot=off  SenseRadDDot=off  SenseAzimDDot=off  SenseDistDDot=off  SenseIncDDot=off
  World Frame : sm_lib/Frames and Transforms/World Frame
  B : PMIOPort  Side=Left
  camera geometry : PMIOPort  Port=2  Side=Left
  y : Outport
  z : Outport  Port=2
  wires:
  PS-Simulink Converter/1 -> y/1
  PS-Simulink Converter1/1 -> z/1
  connections:
  Rigid Transform1/RConn1 -- Rigid Transform2/LConn1
  Rigid Transform2/RConn1 -- Transform Sensor/RConn1 -- File Solid/LConn1
  Rigid Transform/RConn1 -- Rigid Transform1/LConn1
  Transform Sensor/LConn1 -- World Frame/RConn1
  Transform Sensor/RConn2 -- PS-Simulink Converter/LConn1
  B/RConn1 -- Rigid Transform/LConn1
  Transform Sensor/RConn3 -- PS-Simulink Converter1/LConn1
  File Solid/RConn1 -- camera geometry/RConn1

== system twoaxis_camera_gantry_start/	Camera Gantry/contact model ==
  Spatial Contact Force : sm_lib/Forces and Torques/Spatial Contact Force  CoefficientOfDynamicFriction=0.3  CoefficientOfStaticFriction=0.5  SenseContactBaseRotation=off  SenseContactBaseTranslation=off  NormalDamping=1e5  NormalDampingUnits=N/(m/s)  SenseContactFollowerRotation=off  SenseContactFollowerTranslation=off  SenseContactSignal=off  NormalStiffness=1e7  NormalStiffnessUnits=N/m  FrictionalCriticalVelocity=1e-3  FrictionalCriticalVelocityUnits=m/s  ZeroCrossDetectContactStartAndEnd=off  FrictionType=SmoothStickSlip  SenseFrictionalForceMagnitude=off  SenseNormalForceMagnitude=off  NormalForceType=SmoothSpringDamper  SenseNormalVelocity=off  SenseSeparationDistance=off  SenseTangentialVelocity=off  SenseTangentialVelocityMagnitude=off  NormalTransitionRegionWidth=1e-4  NormalTransitionRegionWidthUnits=m
  Spatial Contact Force1 : sm_lib/Forces and Torques/Spatial Contact Force  CoefficientOfDynamicFriction=0.3  CoefficientOfStaticFriction=0.5  SenseContactBaseRotation=off  SenseContactBaseTranslation=off  NormalDamping=1e3  NormalDampingUnits=N/(m/s)  SenseContactFollowerRotation=off  SenseContactFollowerTranslation=off  SenseContactSignal=off  NormalStiffness=1e6  NormalStiffnessUnits=N/m  FrictionalCriticalVelocity=1e-3  FrictionalCriticalVelocityUnits=m/s  ZeroCrossDetectContactStartAndEnd=off  FrictionType=SmoothStickSlip  SenseFrictionalForceMagnitude=off  SenseNormalForceMagnitude=off  NormalForceType=SmoothSpringDamper  SenseNormalVelocity=off  SenseSeparationDistance=off  SenseTangentialVelocity=off  SenseTangentialVelocityMagnitude=off  NormalTransitionRegionWidth=1e-4  NormalTransitionRegionWidthUnits=m
  ceiling : PMIOPort  Side=Left
  wall : PMIOPort  Port=2  Side=Left
  camera : PMIOPort  Port=3  Side=Right
  connections:
  Spatial Contact Force1/LConn1 -- ceiling/RConn1
  Spatial Contact Force1/RConn1 -- Spatial Contact Force/RConn1 -- camera/RConn1
  Spatial Contact Force/LConn1 -- wall/RConn1
